simulink model "QAM16"  (R2024a)
settings: Solver=ode45  StartTime=0.0  StopTime=5000  RelTol=1e-3  EnableMultiTasking=on
PreLoadFcn:
  | QAM16_PreLoadFcn
values from neighbouring files (symbols this model uses):
  chan = [1+j*0.1 .2 j*0.2 0 0 0 0 0 0 0]    [QAM16_PreLoadFcn.m]
  hh = sinc(-3:.25:3)    [QAM16_PreLoadFcn.m]
  k = 9    [QAM16_PreLoadFcn.m]
  k_i0 = (4*theta_0*theta_0)/(1+2*eta*theta_0+theta_0*theta_0)    [QAM16_PreLoadFcn.m]
  k_p0 = (4*eta*theta_0)/(1+2*eta*theta_0+theta_0*theta_0)    [QAM16_PreLoadFcn.m]
  mu = 0.004    [QAM16_PreLoadFcn.m]
undefined symbols (not defined in the file or in its folder): j, QAM, S, vsva2197, xcvc1902, xlipgetpartsetting
libraries: hdlBasic x260, dspmlti4 x2, hdlUtilities x1, hdlDSPIP x1, simulink x1, vmcUtilities x1
(part 1 of 3)
settings Model: Creator=alexc  LastModifiedBy=sdegala
settings SolverCC: AlgebraicLoopSolver=TrustRegion
settings DataIOCC: SaveFormat=Array  SignalLoggingSaveFormat=ModelDataLogs  ReturnWorkspaceOutputs=off  SignalLoggingName=sigsOut
settings OptimizationCC: BlockReduction=off  BooleanDataType=off  DefaultParameterBehavior=Inlined  ExpressionDepthLimit=2147483647  InitFltsAndDblsToZero=on  LifeSpan=inf
settings DebuggingCC: SaveWithParameterizedLinksMsg=none  UnderspecifiedInitializationDetection=Classic  MergeDetectMultiDrivingBlocksExec=none  SignalResolutionControl=TryResolveAllWithWarning  MultiTaskDSMMsg=warning  MultiTaskCondExecSysMsg=none  FcnCallInpInsideContextMsg=warning  UnconnectedInputMsg=warning  UnconnectedOutputMsg=warning  UnconnectedLineMsg=warning  StateNameClashWarn=warning  SFUnexpectedBacktrackingDiag=warning  SFNoUnconditionalDefaultTransitionDiag=warning  SFExecutionAtInitializationDiag=none  ArithmeticOperatorsInVariantConditions=warning
settings HardwareCC: ProdBitPerPointer=32  ProdBitPerSizeT=32  ProdBitPerPtrDiffT=32  ProdLargestAtomicFloat=None  ProdIntDivRoundTo=Undefined  ProdEndianess=Unspecified  ProdWordSize=32  ProdHWDeviceType=32-bit Generic  TargetUnknown=on
settings ModelReferenceCC: EnableRefExpFcnMdlSchedulingChecks=on  PropagateSignalLabelsOutOfModel=off
settings SFSimCC: SimUseLocalCustomCode=off  CustomCodeUndefinedFunction=UseInterfaceOnly
settings RTWCC: RTWUseLocalCustomCode=off  GPUComputeCapability=3.5  DLArmComputeVersion=19.05
settings CodeAppCC: StateflowObjectComments=on
settings GRTTargetCC: TargetFcnLib=ansi_tfl_tmw.mat  TargetLangStandard=C89/C90 (ANSI)  CombineOutputUpdateFcns=off  GRTInterface=on
settings ConfigComp: CovMetricSettings=dw  CovSaveCumulativeToWorkspaceVar=on  CovSaveSingleToWorkspaceVar=on  CovExternalEMLEnable=off

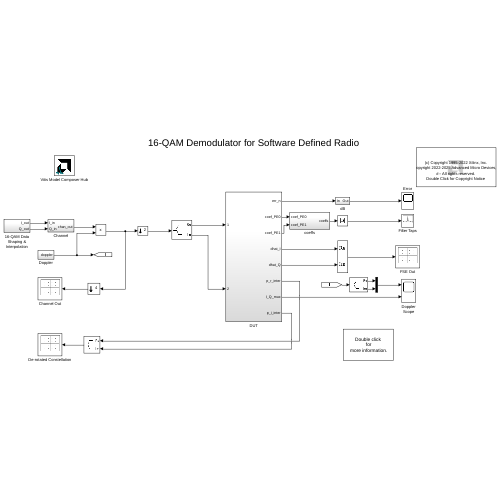
[thumbnail: Simulink's stored preview of the top-level diagram]
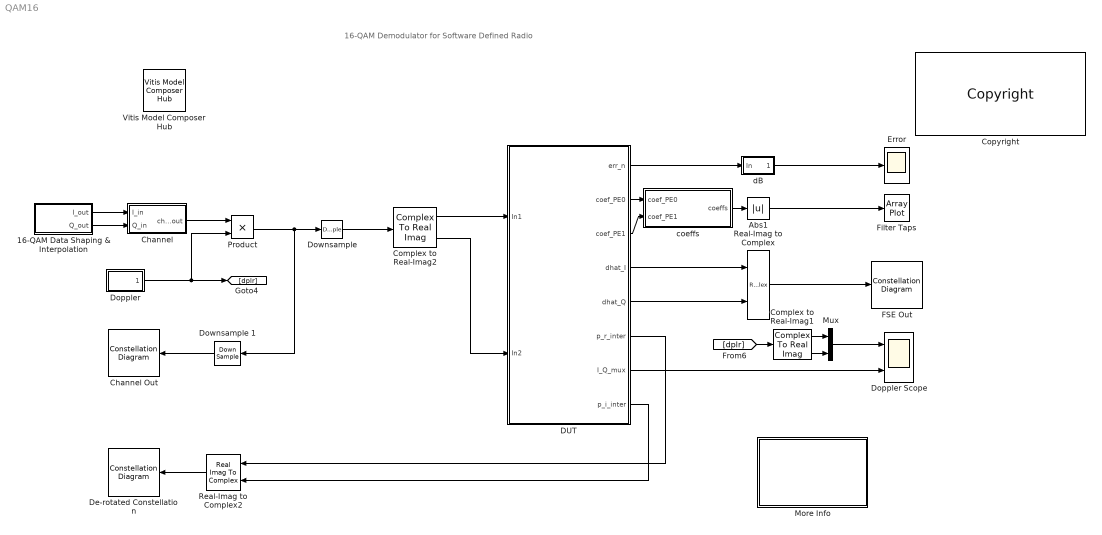
== system QAM16 ==
  note: 16-QAM Demodulator for Software Defined Radio
  16-QAM Data Shaping & Interpolation : Subsystem
  Abs1 : Abs
  Channel : Subsystem
  Channel Out : ConstellationDiagram  WindowPosition=[510.000000,97.000000,342.000000,335.000000,]  Visible=on  ScopeFrameLocation=window  SymbolsToDisplaySource=Property  SymbolsToDisplay=1000  ReferenceConstellation=16-QAM  ShowReferenceConstellation=off  ColorFading=on  DefaultConfigurationName=comm.scopes.ConstellationDiagramBlockCfg
  Complex to Real-Imag1 : ComplexToRealImag
  Complex to Real-Imag2 : ComplexToRealImag
  Copyright : hdlUtilities/Copyright  copyrighttext="(c) Copyright 1995-2022 Xilinx, Inc. <br>(c) Copyright 2022-2025 Advanced Micro Devices, Inc. All rights reserved.<br><br>This document  contains proprietary, confidential information that may be used, copied and/or disclosed only as authorized by a valid licensing agreement with Advanced Micro Devices, Inc. This copyright notice must be retained on all authorized copies.<br><br> This code is provided \"as is\". Advanced Micro Devices, Inc. makes, and the end user receives, no warranties or conditions, express, implied, statutory or otherwise, and Advanced Micro Devices, Inc. specifically disclaims any implied warranties of merchantability, <br>non-infringement, or fitness for a particular purpose."  block_type=copyright
  DUT : Subsystem
  De-rotated Constellation : ConstellationDiagram  WindowPosition=[176.000000,360.000000,339.000000,337.000000,]  Visible=on  ScopeFrameLocation=window  SymbolsToDisplaySource=Property  SymbolsToDisplay=1000  ReferenceConstellation=16-QAM  ColorFading=on  DefaultConfigurationName=comm.scopes.ConstellationDiagramBlockCfg
  Doppler : Subsystem
  Doppler Scope : Scope  NumInputPorts=2
  "Downsample " : DownSample  RateOptions=Allow multirate processing
  Downsample 1 : DownSample  N=4  RateOptions=Allow multirate processing
  Error : Scope
  FSE Out : ConstellationDiagram  WindowPosition=[845.000000,304.000000,340.000000,342.000000,]  Visible=on  ScopeFrameLocation=window  SymbolsToDisplaySource=Property  SymbolsToDisplay=1000  ReferenceConstellation=16-QAM  ShowReferenceConstellation=off  ColorFading=on  DefaultConfigurationName=comm.scopes.ConstellationDiagramBlockCfg
  Filter Taps : ArrayPlot  WindowPosition=[66.000000,260.000000,329.000000,270.000000,]  Visible=on  ScopeFrameLocation=window  PlotType=Line  AxesScaling=Manual  MaximizeAxes=On  XLabel=Samples  YLabel=Filter Coefficients  YLimits=[0.005979,1.0369]  DefaultConfigurationName=dsp.scopes.ArrayPlotBlockSpecification
  More Info : Subsystem
      mask Display: disp('Double click\n for\n more information.')
  Mux : Mux  Inputs=2
  Product : Product  InputSameDT=on  SaturateOnIntegerOverflow=on  OutDataTypeStr=Inherit: Same as first input
  Real-Imag to Complex : RealImagToComplex
  Real-Imag to Complex2 : RealImagToComplex
  Vitis Model Composer Hub : vmcUtilities/Vitis Model Composer Hub  Tag=genX  CodeGeneration=off  SubsystemName=DUT  BlockHierPath=QAM16/DUT  CompilationType=HDLCompilation  SubsystemType=HDLNode  ExportTypeV2=IP Catalog  StartColumn=1  NumberOfColumns=1  TargetDirectory=./netlist  exportDesign=on  analyzeDesign=off  validateDesignOnHw=off  ExportType=System Generator  IpVendor=xilinx.com  IpLibrary=hls  IpVersion=1.0  IpHWLanguage=Verilog  AieCompilerOptions={}  AieSimulatorOptions={}  CreateTestbench=off  TestbenchStackSize=10  RunRtlSim=off  RunCSim=off  RunAieSim=off  AieSimTimeout=50000  RunAieSimProfiling=off  LaunchVitisAnalyzer=off  PlotOutput=off  RunX86Sim=off  X86SimTimeout=10  GenHwImage=off  GenLibadfXo=on  GenHwValidationCode=off  PlatformType=Not Specified  HwSystemType=Baremetal  HwValidationTarget=hw  ProjDevice=xcvc1902-vsva2197-1LP-e-S  ProjDevicePart=xcvc1902-vsva2197-1LP-e-S  AIEType=AIE  SamplePeriod=-1  ClockFrequency=200  DataPathParallelism=1  xilinxfamily=versalaicore  part=xcvc1902  speed=-1LP-e-S  package=vsva2197  directory=./netlist/ip/DUT/src  testbench=off  incr_netlist=off  synthesis_tool=Vivado  clock_wrapper=Clock Enables  dbl_ovrd=According to Block Masks  dcm_input_clock_period=10  sysclk_period=10  simulink_period=1  eval_field=0  IPInfoJsonString="{\"DUTSubsystemName\":\"DUT\",\"HDLSubsystem\":{\"SubsystemName\":\"DUT\",\"IPName\":\"DUT\",\"IPLibrary\":\"VMC\",\"IPVendor\":\"User Company\",\"IPVersion\":\"1.0\",\"TargetDirectory\":\"./netlist\",\"SubsystemDir\":\"./netlist/ip/DUT\",\"FreqHz\":\"100000000\"},\"SubsystemTag\":\"HDLNode\"}"  LogFileName=/proj/xhdhdstaff5/sdegala/Head1/HEAD/ModelComposer_Sept16/Vitis_Model_Composer/Examples/HDL/Digital_Communications/16_QAM_demodulator/netlist/model_composer.log  NThreads=4  IPConfigFile=/tmp/vmctmp-9769773316677438567/QAM16_ipconfig.json
  coeffs : Subsystem
  dB : Subsystem
  wires:
  [dplr] -> Complex to Real-Imag1/1
  Complex to Real-Imag2/1 -> DUT/1(In1)
  Abs1/1 -> Filter Taps/1
  DUT/8(p_i_inter) -> Real-Imag to Complex2/2
  dB/1(Out) -> Error/1
  16-QAM Data Shaping & Interpolation/2(Q_out) -> Channel/2(Q_in)
  Mux/1 -> Doppler Scope/1
  DUT/4(dhat_I) -> Real-Imag to Complex/1
  Channel/1(chan_out) -> Product/1
  DUT/6(p_r_inter) -> Real-Imag to Complex2/1
  Downsample 1/1 -> Channel Out/1
  DUT/1(err_n) -> dB/1(In)
  Real-Imag to Complex2/1 -> De-rotated Constellation/1
  Complex to Real-Imag1/2 -> Mux/2
  16-QAM Data Shaping & Interpolation/1(I_out) -> Channel/1(I_in)
  DUT/5(dhat_Q) -> Real-Imag to Complex/2
  Complex to Real-Imag2/2 -> DUT/2(In2)
  Complex to Real-Imag1/1 -> Mux/1
  Real-Imag to Complex/1 -> FSE Out/1
  Doppler/1(doppler) -> Product/2, [dplr]
  Product/1 -> "Downsample "/1, Downsample 1/1
  "Downsample "/1 -> Complex to Real-Imag2/1
  DUT/7(I_Q_mux) -> Doppler Scope/2
  DUT/2(coef_PE0) -> coeffs/1(coef_PE0)
  coeffs/1(coeffs) -> Abs1/1
  DUT/3(coef_PE1) -> coeffs/2(coef_PE1)

== system QAM16/16-QAM Data Shaping & Interpolation ==
  Complex to Real-Imag5 : ComplexToRealImag
  "FIR Interpolation " : dspmlti4/FIR Interpolation  FilterSource=Dialog parameters  PrivateCoeffs=0  h=[hh]  L=4  FilterObject=Hm_firinterp  framing=Allow multirate processing  outputBufInitCond=0  roundingMode=Floor  overflowMode=off  firstCoeffDataTypeStr=Inherit: Same word length as input  firstCoeffMin=[]  firstCoeffMax=[]  firstCoeffLastDataTypeStr=Inherit: Same word length as input  outputDataTypeStr=Inherit: Same as accumulator  outputMin=[]  outputMax=[]  outputLastDataTypeStr=Inherit: Same as accumulator
  FIR Interpolation 1 : dspmlti4/FIR Interpolation  FilterSource=Dialog parameters  PrivateCoeffs=0  h=[hh]  L=4  FilterObject=Hm_firinterp  framing=Allow multirate processing  outputBufInitCond=0  roundingMode=Floor  overflowMode=off  firstCoeffDataTypeStr=Inherit: Same word length as input  firstCoeffMin=[]  firstCoeffMax=[]  firstCoeffLastDataTypeStr=Inherit: Same word length as input  outputDataTypeStr=Inherit: Same as accumulator  outputMin=[]  outputMax=[]  outputLastDataTypeStr=Inherit: Same as accumulator
  QAM16 Source : Subsystem
  I_out : Outport  VectorParamsAs1DForOutWhenUnconnected=off
  Q_out : Outport  Port=2  VectorParamsAs1DForOutWhenUnconnected=off
  wires:
  Complex to Real-Imag5/1 -> "FIR Interpolation "/1
  Complex to Real-Imag5/2 -> FIR Interpolation 1/1
  QAM16 Source/1(random_data) -> Complex to Real-Imag5/1
  "FIR Interpolation "/1 -> I_out/1
  FIR Interpolation 1/1 -> Q_out/1

== system QAM16/Channel ==
  I_in : Inport
  Q_in : Inport  Port=2
  Channel : Subsystem
  Channel1 : Subsystem
  Gain : Gain  Gain=j  SaturateOnIntegerOverflow=on  OutDataTypeStr=Inherit: Same as input  ParamDataTypeStr=Inherit: Same as input
  Sum : Sum  InputSameDT=on  SaturateOnIntegerOverflow=on  OutDataTypeStr=Inherit: Same as first input
  chan_out : Outport  VectorParamsAs1DForOutWhenUnconnected=off
  wires:
  Gain/1 -> Sum/2
  Channel/1(y_n) -> Sum/1
  Channel1/1(y_n) -> Gain/1
  I_in/1 -> Channel/1(x_n)
  Q_in/1 -> Channel1/1(x_n)
  Sum/1 -> chan_out/1

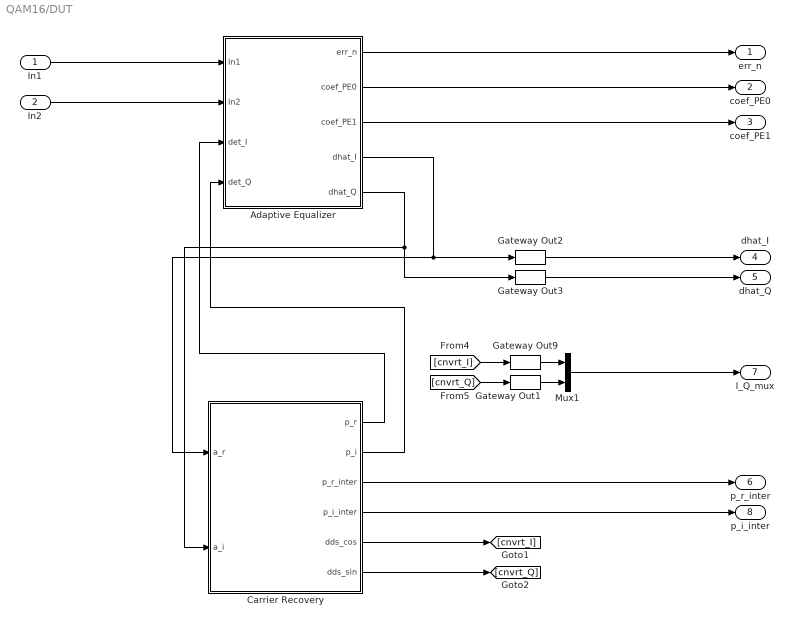
== system QAM16/DUT ==
  In1 : Inport
  In2 : Inport  Port=2
  Adaptive Equalizer : Subsystem
  Carrier Recovery : Subsystem
  Gateway Out{1..3,9} (4 alike) : hdlBasic/Gateway Out  inherit_from_input=off  bool_to_boolean=off  hdl_port=off  rows=1  columns=1  UseAsDAC=off  DACChannel='1'  interface=None  automatic_assignment=on  address_offset=hex2dec('00')  intf_name=''  intf_description=''  timing_constraint=None  locs_specified=off  LOCs={}  io_standard={}  XmcBlockStatus=1  maskContainerNames=group4  block_type=gatewayout  block_config=sysgen:gateway_out_config  block_width_w=590  block_height_w=620  block_width=620  block_height=750
  Mux1 : Mux  Inputs=2
  err_n : Outport
  coef_PE0 : Outport  Port=2
  coef_PE1 : Outport  Port=3
  dhat_I : Outport  Port=4
  dhat_Q : Outport  Port=5
  p_r_inter : Outport  Port=6
  I_Q_mux : Outport  Port=7
  p_i_inter : Outport  Port=8
  wires:
  In1/1 -> Adaptive Equalizer/1(In1)
  Gateway Out1/1 -> Mux1/2
  Carrier Recovery/4(p_i_inter) -> p_i_inter/1
  Adaptive Equalizer/2(coef_PE0) -> coef_PE0/1
  Adaptive Equalizer/1(err_n) -> err_n/1
  In2/1 -> Adaptive Equalizer/2(In2)
  Gateway Out3/1 -> dhat_Q/1
  Mux1/1 -> I_Q_mux/1
  Carrier Recovery/2(p_i) -> Adaptive Equalizer/4(det_Q)
  Carrier Recovery/5(dds_cos) -> [cnvrt_I]
  Adaptive Equalizer/5(dhat_Q) -> Gateway Out3/1, Carrier Recovery/2(a_i)
  Carrier Recovery/3(p_r_inter) -> p_r_inter/1
  Gateway Out9/1 -> Mux1/1
  [cnvrt_Q] -> Gateway Out1/1
  Carrier Recovery/6(dds_sin) -> [cnvrt_Q]
  Adaptive Equalizer/4(dhat_I) -> Gateway Out2/1, Carrier Recovery/1(a_r)
  [cnvrt_I] -> Gateway Out9/1
  Carrier Recovery/1(p_r) -> Adaptive Equalizer/3(det_I)
  Gateway Out2/1 -> dhat_I/1
  Adaptive Equalizer/3(coef_PE1) -> coef_PE1/1

== system QAM16/Doppler ==
  DSP Constant : Constant  VectorParams1D=off  SampleTime=1
  Frequency Delta : simulink/Math Operations/Slider Gain  gain=0.001  low=-0.1  high=0.1
  R:I : RealImagToComplex
  TX Doppler : Subsystem
  Terminator : Terminator
  doppler : Outport  VectorParamsAs1DForOutWhenUnconnected=off
  wires:
  TX Doppler/1(Cos) -> R:I/1
  TX Doppler/2(Sin) -> R:I/2
  Frequency Delta/1 -> TX Doppler/1(In1)
  DSP Constant/1 -> Frequency Delta/1
  R:I/1 -> doppler/1
  TX Doppler/3(DDS Theta) -> Terminator/1

== system QAM16/More Info ==
  note: 16-QAM Demodulator for Software Defined Radio
  note: This design implements an equalized 16-QAM demodulator for use in a software defined
      | radio.  The receiver architecture provides subsystems that demonstrate adaptive channel
      | equalization and carrier tracking on a random QAM data source.
      |
      | In addition to Vitis Model Composer demodulator components, the model includes Simulink
      | subsystems that introduce channel effects and Doppler content into the data source.  Scopes
      | are provided at important nodes for analysis purposes.  The operation of receiver is best
      | illustrated with a long simulation duration, so that the points in the de-rotated constellation
      | have sufficient time to converge.
      |
      | Additional information on software radios can be found at:
      |
      | Chris H. Dick, "Design and implementation of high-performance FPGA signal processing
      | datapaths for software-defined radios" VMEbus Systems, August 2001

== system QAM16/coeffs ==
  note: The equalizer ALU divides the processing between two
      | polyphase arms.  each with their own PE.  The four filter
      | operations are scheduled onto a single complex multiply
      | -accumulate (MAC) engine.  Similarly, the 4 coefficient
      | updates are folded onto a single LMS PE.
  coef_PE0 : Inport
  coef_PE1 : Inport  Port=2
  Buffer : Buffer  N=8
  Discrete Pulse Generator : DiscretePulseGenerator  SampleTime=.5
  Switch1 : Switch  Threshold=.5
  coeffs : Outport
  wires:
  coef_PE0/1 -> Switch1/3
  coef_PE1/1 -> Switch1/1
  Discrete Pulse Generator/1 -> Switch1/2
  Switch1/1 -> Buffer/1
  Buffer/1 -> coeffs/1

== system QAM16/dB ==
  In : Inport
  Abs : Abs
  Constant : Constant  Value=0
  Constant1 : Constant
  Constant2 : Constant
  Gain1 : Gain  Gain=20  SaturateOnIntegerOverflow=on  OutDataTypeStr=Inherit: Same as input  ParamDataTypeStr=Inherit: Same as input
  Multiport Switch : MultiPortSwitch  Inputs=2
  Relational Operator : RelationalOperator  Operator===
  Sum : Sum  Inputs=|++  InputSameDT=on  SaturateOnIntegerOverflow=on  OutDataTypeStr=Inherit: Same as first input
  log10 : Math  Operator=log10  SignedPower=on
  Out : Outport  VectorParamsAs1DForOutWhenUnconnected=off
  wires:
  Multiport Switch/1 -> log10/1
  Constant1/1 -> Multiport Switch/3
  Constant/1 -> Relational Operator/1
  Abs/1 -> Multiport Switch/2, Relational Operator/2
  Constant2/1 -> Sum/2
  Sum/1 -> Multiport Switch/1
  Relational Operator/1 -> Sum/1
  Gain1/1 -> Out/1
  In/1 -> Abs/1
  log10/1 -> Gain1/1

== system QAM16/16-QAM Data Shaping & Interpolation/QAM16 Source ==
  QAM16 - I : Subsystem
  QAM16 -Q : Subsystem
  Real-Imag to Complex : RealImagToComplex
  random_data : Outport  VectorParamsAs1DForOutWhenUnconnected=off
  wires:
  Real-Imag to Complex/1 -> random_data/1
  QAM16 -Q/1(Q) -> Real-Imag to Complex/2
  QAM16 - I/1(I) -> Real-Imag to Complex/1

== system QAM16/Channel/Channel ==
  x_n : Inport
  Channel Response : Subsystem
  y_n : Outport  VectorParamsAs1DForOutWhenUnconnected=off
  wires:
  Channel Response/1(y_n) -> y_n/1
  x_n/1 -> Channel Response/1(x_n)

== system QAM16/Channel/Channel1 ==
  x_n : Inport
  Channel Response : Subsystem
  y_n : Outport  VectorParamsAs1DForOutWhenUnconnected=off
  wires:
  Channel Response/1(y_n) -> y_n/1
  x_n/1 -> Channel Response/1(x_n)

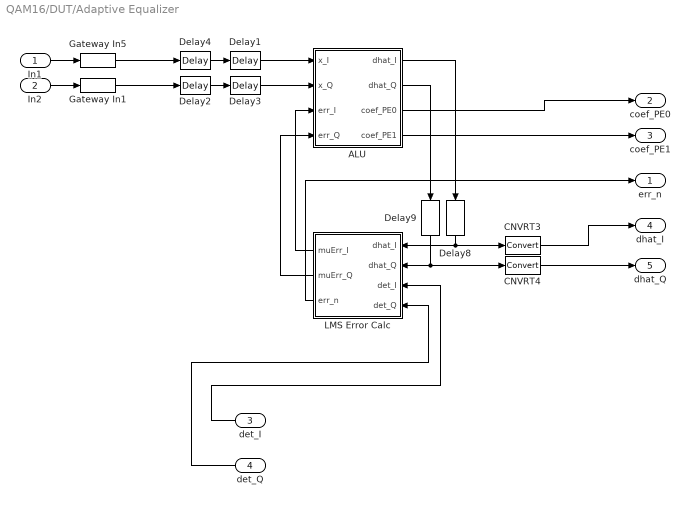
== system QAM16/DUT/Adaptive Equalizer ==
  In1 : Inport
  In2 : Inport  Port=2
  det_I : Inport  Port=3
  det_Q : Inport  Port=4
  ALU : Subsystem
  CNVRT3 : hdlBasic/Convert  gui_display_data_type=Fixed-point  arith_type=Signed (2's comp)  n_bits=18  bin_pt=14  float_type=Single  exp_bits=8  fraction_bits=24  quantization="Round  (unbiased: +/- Inf)"  overflow=Wrap  en=off  latency=0  pipeline=off  XmcBlockStatus=1  maskContainerNames=group2  block_type=convert  block_config=sysgen:Convert_config  block_width=595  block_height=885
  CNVRT4 : hdlBasic/Convert  gui_display_data_type=Fixed-point  arith_type=Signed (2's comp)  n_bits=18  bin_pt=14  float_type=Single  exp_bits=8  fraction_bits=24  quantization="Round  (unbiased: +/- Inf)"  overflow=Wrap  en=off  latency=0  pipeline=off  XmcBlockStatus=1  maskContainerNames=group2  block_type=convert  block_config=sysgen:Convert_config  block_width=595  block_height=885
  Delay{1..4} (4 alike) : hdlBasic/Delay  rst=off  en=off  latency=1  reg_retiming=off  XmcBlockStatus=1  maskContainerNames=group1  block_type=delay  block_config=sysgen:Delay_config
  Delay8 : hdlBasic/Delay  rst=off  en=off  latency=k-7  reg_retiming=off  XmcBlockStatus=1  maskContainerNames=group1  block_type=delay  block_config=sysgen:Delay_config
  Delay9 : hdlBasic/Delay  rst=off  en=off  latency=k-7  reg_retiming=off  XmcBlockStatus=1  maskContainerNames=group1  block_type=delay  block_config=sysgen:Delay_config
  Gateway In1 : hdlBasic/Gateway In  gui_display_data_type=Fixed-point  arith_type=Signed (2's comp)  n_bits=xn_ni  bin_pt=xn_nf  preci_type=Single  exp_width=8  frac_width=24  rows=1  columns=1  quantization="Round  (unbiased: +/- Inf)"  overflow=Saturate  period=2  UseAsADC=off  ADCChannel='1'  interface=None  automatic_assignment=on  address_offset=hex2dec('00')  intf_name=''  intf_description=''  default_value=0  timing_constraint=None  locs_specified=off  LOCs={}  io_standard={}  inherit_from_input=off  hdl_port=on  XmcBlockStatus=1  maskContainerNames=group4  block_type=gatewayin  block_config=sysgen:gateway_in_config  block_width_w=590  block_height_w=620  block_width=640  block_height=850
  Gateway In5 : hdlBasic/Gateway In  gui_display_data_type=Fixed-point  arith_type=Signed (2's comp)  n_bits=xn_ni  bin_pt=xn_nf  preci_type=Single  exp_width=8  frac_width=24  rows=1  columns=1  quantization="Round  (unbiased: +/- Inf)"  overflow=Saturate  period=2  UseAsADC=off  ADCChannel='1'  interface=None  automatic_assignment=on  address_offset=hex2dec('00')  intf_name=''  intf_description=''  default_value=0  timing_constraint=None  locs_specified=off  LOCs={}  io_standard={}  inherit_from_input=off  hdl_port=on  XmcBlockStatus=1  maskContainerNames=group4  block_type=gatewayin  block_config=sysgen:gateway_in_config  block_width_w=590  block_height_w=620  block_width=640  block_height=850
  LMS Error Calc : Subsystem
  err_n : Outport
  coef_PE0 : Outport  Port=2
  coef_PE1 : Outport  Port=3
  dhat_I : Outport  Port=4
  dhat_Q : Outport  Port=5
  wires:
  ALU/2(dhat_Q) -> Delay9/1
  ALU/3(coef_PE0) -> coef_PE0/1
  det_I/1 -> LMS Error Calc/3(det_I)
  LMS Error Calc/3(err_n) -> err_n/1
  Delay9/1 -> LMS Error Calc/2(dhat_Q), CNVRT4/1
  In2/1 -> Gateway In1/1
  det_Q/1 -> LMS Error Calc/4(det_Q)
  CNVRT3/1 -> dhat_I/1
  In1/1 -> Gateway In5/1
  Delay2/1 -> Delay3/1
  Delay3/1 -> ALU/2(x_Q)
  Gateway In5/1 -> Delay4/1
  ALU/1(dhat_I) -> Delay8/1
  Delay8/1 -> LMS Error Calc/1(dhat_I), CNVRT3/1
  Delay1/1 -> ALU/1(x_I)
  LMS Error Calc/2(muErr_Q) -> ALU/4(err_Q)
  LMS Error Calc/1(muErr_I) -> ALU/3(err_I)
  CNVRT4/1 -> dhat_Q/1
  Gateway In1/1 -> Delay2/1
  Delay4/1 -> Delay1/1
  ALU/4(coef_PE1) -> coef_PE1/1

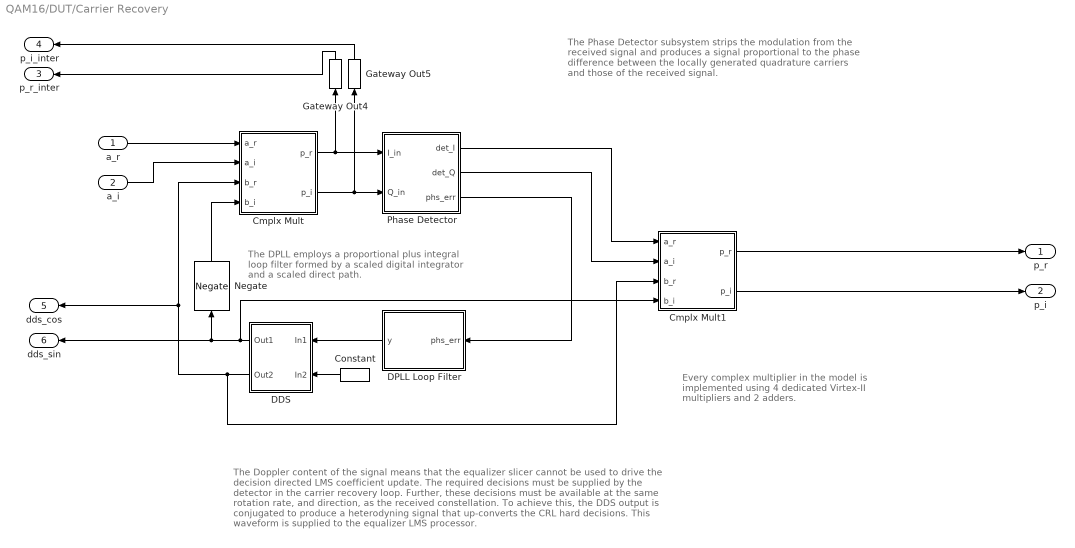
== system QAM16/DUT/Carrier Recovery ==
  note: The DPLL employs a proportional plus integral
      | loop filter formed by a scaled digital integrator
      | and a scaled direct path.
  note: The Phase Detector subsystem strips the modulation
      | from the received signal and produces a signal proportional
      | to the phase difference between the locally generated
      | quadrature carriers and those of the received signal.
  note: The Doppler content of the signal means that the equalizer slicer cannot be used
      | to drive the decision directed LMS coefficient update.  The required decisions must
      | be supplied by the detector in the carrier recovery loop.  Further, these decisions
      | must be available at the same rotation rate, and direction, as the received constellation.
      | To achieve this, the DDS output is conjugated to produce a heterodyning signal
      | that up-converts the CRL hard decisions. This waveform is supplied to the equalizer
      | LMS processor.
  note: Every complex multiplier in the model is
      | implemented using 4 dedicated Virtex-II
      | multipliers and 2 adders.
  a_r : Inport
  a_i : Inport  Port=2
  Cmplx Mult : Subsystem
  Cmplx Mult1 : Subsystem
  Constant : hdlBasic/Constant  const=1  gui_display_data_type=Boolean  arith_type=Boolean  n_bits=1  bin_pt=0  preci_type=Single  exp_width=8  frac_width=24  explicit_period=off  period=1  XmcBlockStatus=1  maskContainerNames=tabcontainer1  block_type=constant  block_config=sysgen:Constant_config
  DDS : Subsystem
  DPLL Loop Filter : Subsystem
  Gateway Out4 : hdlBasic/Gateway Out  inherit_from_input=off  bool_to_boolean=off  hdl_port=on  rows=1  columns=1  UseAsDAC=off  DACChannel='1'  interface=None  automatic_assignment=on  address_offset=hex2dec('00')  intf_name=''  intf_description=''  timing_constraint="Data Rate;  Set 'FAST' Attribute"  locs_specified=off  LOCs={}  io_standard={}  XmcBlockStatus=1  maskContainerNames=group4  block_type=gatewayout  block_config=sysgen:gateway_out_config  block_width_w=590  block_height_w=620  block_width=620  block_height=750
  Gateway Out5 : hdlBasic/Gateway Out  inherit_from_input=off  bool_to_boolean=off  hdl_port=on  rows=1  columns=1  UseAsDAC=off  DACChannel='1'  interface=None  automatic_assignment=on  address_offset=hex2dec('00')  intf_name=''  intf_description=''  timing_constraint="Data Rate;  Set 'FAST' Attribute"  locs_specified=off  LOCs={}  io_standard={}  XmcBlockStatus=1  maskContainerNames=group4  block_type=gatewayout  block_config=sysgen:gateway_out_config  block_width_w=590  block_height_w=620  block_width=620  block_height=750
  Negate : hdlBasic/Negate  precision=Full  arith_type=Unsigned  n_bits=8  bin_pt=2  quantization=Truncate  overflow=Wrap  en=off  latency=0  XmcBlockStatus=1  maskContainerNames=tabcontainer1  block_type=negate  block_config=sysgen:Negate_config
  Phase Detector : Subsystem
  p_r : Outport
  p_i : Outport  Port=2
  p_r_inter : Outport  Port=3
  p_i_inter : Outport  Port=4
  dds_cos : Outport  Port=5
  dds_sin : Outport  Port=6
  wires:
  DPLL Loop Filter/1(y) -> DDS/1(In1)
  Negate/1 -> Cmplx Mult/4(b_i)
  Cmplx Mult/1(p_r) -> Gateway Out4/1, Phase Detector/1(I_in)
  Cmplx Mult1/2(p_i) -> p_i/1
  a_r/1 -> Cmplx Mult/1(a_r)
  DDS/2(Out2) -> dds_cos/1, Cmplx Mult/3(b_r), Cmplx Mult1/3(b_r)
  Gateway Out5/1 -> p_i_inter/1
  Constant/1 -> DDS/2(In2)
  a_i/1 -> Cmplx Mult/2(a_i)
  DDS/1(Out1) -> Negate/1, dds_sin/1, Cmplx Mult1/4(b_i)
  Cmplx Mult1/1(p_r) -> p_r/1
  Phase Detector/3(phs_err) -> DPLL Loop Filter/1(phs_err)
  Phase Detector/2(det_Q) -> Cmplx Mult1/2(a_i)
  Cmplx Mult/2(p_i) -> Gateway Out5/1, Phase Detector/2(Q_in)
  Phase Detector/1(det_I) -> Cmplx Mult1/1(a_r)
  Gateway Out4/1 -> p_r_inter/1

== system QAM16/Doppler/TX Doppler ==
  In1 : Inport
  Sum5 : Sum  Inputs=|++  InputSameDT=on  SaturateOnIntegerOverflow=on  OutDataTypeStr=Inherit: Same as first input
  Trigonometric Function1 : Trigonometry  Operator=cos
  Trigonometric Function2 : Trigonometry
  Unit Delay2 : UnitDelay  HasFrameUpgradeWarning=on
  c2 : Gain  Gain=2*pi  SaturateOnIntegerOverflow=on  OutDataTypeStr=Inherit: Same as input  ParamDataTypeStr=Inherit: Same as input
  c3 : Gain  SaturateOnIntegerOverflow=on  OutDataTypeStr=Inherit: Same as input  ParamDataTypeStr=Inherit: Same as input
  Cos : Outport  VectorParamsAs1DForOutWhenUnconnected=off
  Sin : Outport  Port=2  VectorParamsAs1DForOutWhenUnconnected=off
  DDS Theta : Outport  Port=3  VectorParamsAs1DForOutWhenUnconnected=off
  wires:
  c2/1 -> Trigonometric Function1/1, Trigonometric Function2/1, DDS Theta/1
  Sum5/1 -> Unit Delay2/1
  Unit Delay2/1 -> c2/1, Sum5/2
  Trigonometric Function2/1 -> c3/1
  c3/1 -> Sin/1
  Trigonometric Function1/1 -> Cos/1
  In1/1 -> Sum5/1

== system QAM16/16-QAM Data Shaping & Interpolation/QAM16 Source/QAM16 - I ==
  Constant : Constant  Value=3
  Gain : Gain  Gain=2  SaturateOnIntegerOverflow=on  OutDataTypeStr=Inherit: Same as input  ParamDataTypeStr=Inherit: Same as input
  Gain1 : Gain  Gain=1/3  SaturateOnIntegerOverflow=on  OutDataTypeStr=Inherit: Same as input  ParamDataTypeStr=Inherit: Same as input
  Random Integer Generator : Subsystem  mask{M=4, seed=11, Ts=4}
      mask prompts: M "M-ary Number"; seed "Initial seed"; Ts "Sample Time"
  Sum : Sum  Inputs=|+-  InputSameDT=on  SaturateOnIntegerOverflow=on  OutDataTypeStr=Inherit: Same as first input
  I : Outport  VectorParamsAs1DForOutWhenUnconnected=off
  wires:
  Gain1/1 -> I/1
  Sum/1 -> Gain1/1
  Constant/1 -> Sum/2
  Gain/1 -> Sum/1
  Random Integer Generator/1(Out1) -> Gain/1

== system QAM16/16-QAM Data Shaping & Interpolation/QAM16 Source/QAM16 -Q ==
  Constant : Constant  Value=3
  Gain : Gain  Gain=2  SaturateOnIntegerOverflow=on  OutDataTypeStr=Inherit: Same as input  ParamDataTypeStr=Inherit: Same as input
  Gain1 : Gain  Gain=1/3  SaturateOnIntegerOverflow=on  OutDataTypeStr=Inherit: Same as input  ParamDataTypeStr=Inherit: Same as input
  Random Integer Generator : Subsystem  mask{M=4, seed=72, Ts=4}
      mask prompts: M "M-ary Number"; seed "Initial seed"; Ts "Sample Time"
  Sum : Sum  Inputs=|+-  InputSameDT=on  SaturateOnIntegerOverflow=on  OutDataTypeStr=Inherit: Same as first input
  Q : Outport  VectorParamsAs1DForOutWhenUnconnected=off
  wires:
  Gain1/1 -> Q/1
  Sum/1 -> Gain1/1
  Constant/1 -> Sum/2
  Gain/1 -> Sum/1
  Random Integer Generator/1(Out1) -> Gain/1

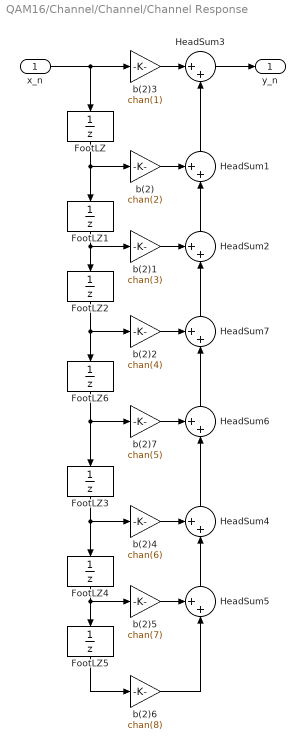
== system QAM16/Channel/Channel/Channel Response ==
  x_n : Inport
  FootLZ : UnitDelay  HasFrameUpgradeWarning=on
  FootLZ{1..2,4..6} (5 alike) : UnitDelay  SampleTime=-1  HasFrameUpgradeWarning=on
  FootLZ3 : UnitDelay  HasFrameUpgradeWarning=on
  HeadSum{1..2,4..7} (6 alike) : Sum  Inputs=++|  InputSameDT=on  SaturateOnIntegerOverflow=on  OutDataTypeStr=Inherit: Same as first input
  HeadSum3 : Sum  Inputs=|++  InputSameDT=on  SaturateOnIntegerOverflow=on  OutDataTypeStr=Inherit: Same as first input
  b(2) : Gain  Gain=chan(2)  SaturateOnIntegerOverflow=on  OutDataTypeStr=Inherit: Same as input  ParamDataTypeStr=Inherit: Same as input
  b(2)1 : Gain  Gain=chan(3)  SaturateOnIntegerOverflow=on  OutDataTypeStr=Inherit: Same as input  ParamDataTypeStr=Inherit: Same as input
  b(2)2 : Gain  Gain=chan(4)  SaturateOnIntegerOverflow=on  OutDataTypeStr=Inherit: Same as input  ParamDataTypeStr=Inherit: Same as input
  b(2)3 : Gain  Gain=chan(1)  SaturateOnIntegerOverflow=on  OutDataTypeStr=Inherit: Same as input  ParamDataTypeStr=Inherit: Same as input
  b(2)4 : Gain  Gain=chan(6)  SaturateOnIntegerOverflow=on  OutDataTypeStr=Inherit: Same as input  ParamDataTypeStr=Inherit: Same as input
  b(2)5 : Gain  Gain=chan(7)  SaturateOnIntegerOverflow=on  OutDataTypeStr=Inherit: Same as input  ParamDataTypeStr=Inherit: Same as input
  b(2)6 : Gain  Gain=chan(8)  SaturateOnIntegerOverflow=on  OutDataTypeStr=Inherit: Same as input  ParamDataTypeStr=Inherit: Same as input
  b(2)7 : Gain  Gain=chan(5)  SaturateOnIntegerOverflow=on  OutDataTypeStr=Inherit: Same as input  ParamDataTypeStr=Inherit: Same as input
  y_n : Outport  VectorParamsAs1DForOutWhenUnconnected=off
  wires:
  HeadSum3/1 -> y_n/1
  HeadSum1/1 -> HeadSum3/2
  b(2)3/1 -> HeadSum3/1
  x_n/1 -> b(2)3/1, FootLZ/1
  HeadSum2/1 -> HeadSum1/2
  b(2)1/1 -> HeadSum2/1
  b(2)/1 -> HeadSum1/1
  FootLZ1/1 -> b(2)1/1, FootLZ2/1
  FootLZ/1 -> FootLZ1/1, b(2)/1
  FootLZ2/1 -> b(2)2/1, FootLZ6/1
  b(2)7/1 -> HeadSum6/1
  b(2)6/1 -> HeadSum5/2
  HeadSum5/1 -> HeadSum4/2
  b(2)5/1 -> HeadSum5/1
  b(2)4/1 -> HeadSum4/1
  FootLZ5/1 -> b(2)6/1
  FootLZ4/1 -> b(2)5/1, FootLZ5/1
  FootLZ3/1 -> FootLZ4/1, b(2)4/1
  FootLZ6/1 -> b(2)7/1, FootLZ3/1
  b(2)2/1 -> HeadSum7/1
  HeadSum7/1 -> HeadSum2/2
  HeadSum4/1 -> HeadSum6/2
  HeadSum6/1 -> HeadSum7/2

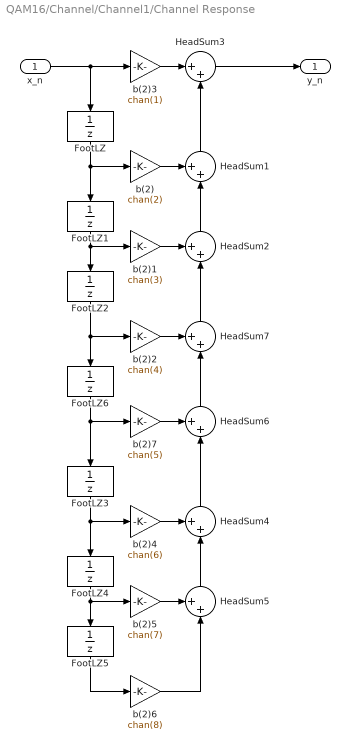
== system QAM16/Channel/Channel1/Channel Response ==
  x_n : Inport
  FootLZ : UnitDelay  HasFrameUpgradeWarning=on
  FootLZ{1..2,4..6} (5 alike) : UnitDelay  SampleTime=-1  HasFrameUpgradeWarning=on
  FootLZ3 : UnitDelay  HasFrameUpgradeWarning=on
  HeadSum{1..2,4..7} (6 alike) : Sum  Inputs=++|  InputSameDT=on  SaturateOnIntegerOverflow=on  OutDataTypeStr=Inherit: Same as first input
  HeadSum3 : Sum  Inputs=|++  InputSameDT=on  SaturateOnIntegerOverflow=on  OutDataTypeStr=Inherit: Same as first input
  b(2) : Gain  Gain=chan(2)  SaturateOnIntegerOverflow=on  OutDataTypeStr=Inherit: Same as input  ParamDataTypeStr=Inherit: Same as input
  b(2)1 : Gain  Gain=chan(3)  SaturateOnIntegerOverflow=on  OutDataTypeStr=Inherit: Same as input  ParamDataTypeStr=Inherit: Same as input
  b(2)2 : Gain  Gain=chan(4)  SaturateOnIntegerOverflow=on  OutDataTypeStr=Inherit: Same as input  ParamDataTypeStr=Inherit: Same as input
  b(2)3 : Gain  Gain=chan(1)  SaturateOnIntegerOverflow=on  OutDataTypeStr=Inherit: Same as input  ParamDataTypeStr=Inherit: Same as input
  b(2)4 : Gain  Gain=chan(6)  SaturateOnIntegerOverflow=on  OutDataTypeStr=Inherit: Same as input  ParamDataTypeStr=Inherit: Same as input
  b(2)5 : Gain  Gain=chan(7)  SaturateOnIntegerOverflow=on  OutDataTypeStr=Inherit: Same as input  ParamDataTypeStr=Inherit: Same as input
  b(2)6 : Gain  Gain=chan(8)  SaturateOnIntegerOverflow=on  OutDataTypeStr=Inherit: Same as input  ParamDataTypeStr=Inherit: Same as input
  b(2)7 : Gain  Gain=chan(5)  SaturateOnIntegerOverflow=on  OutDataTypeStr=Inherit: Same as input  ParamDataTypeStr=Inherit: Same as input
  y_n : Outport  VectorParamsAs1DForOutWhenUnconnected=off
  wires:
  HeadSum3/1 -> y_n/1
  HeadSum1/1 -> HeadSum3/2
  b(2)3/1 -> HeadSum3/1
  x_n/1 -> b(2)3/1, FootLZ/1
  HeadSum2/1 -> HeadSum1/2
  b(2)1/1 -> HeadSum2/1
  b(2)/1 -> HeadSum1/1
  FootLZ1/1 -> b(2)1/1, FootLZ2/1
  FootLZ/1 -> FootLZ1/1, b(2)/1
  HeadSum4/1 -> HeadSum6/2
  b(2)7/1 -> HeadSum6/1
  b(2)6/1 -> HeadSum5/2
  HeadSum5/1 -> HeadSum4/2
  b(2)5/1 -> HeadSum5/1
  b(2)4/1 -> HeadSum4/1
  FootLZ5/1 -> b(2)6/1
  FootLZ4/1 -> b(2)5/1, FootLZ5/1
  FootLZ3/1 -> FootLZ4/1, b(2)4/1
  FootLZ2/1 -> b(2)2/1, FootLZ6/1
  FootLZ6/1 -> FootLZ3/1, b(2)7/1
  HeadSum6/1 -> HeadSum7/2
  HeadSum7/1 -> HeadSum2/2
  b(2)2/1 -> HeadSum7/1

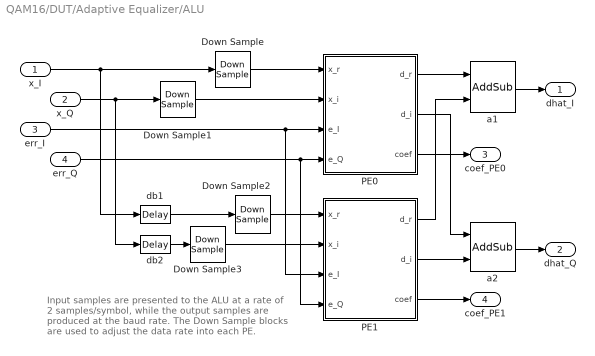
== system QAM16/DUT/Adaptive Equalizer/ALU ==
  note: Input samples are presented to the ALU at a rate
      | of 2 samples/symbol, while the output samples
      | are produced at the baud rate.  The Down
      | Sample blocks are used to adjust the data rate
      | into each PE.
  x_I : Inport
  x_Q : Inport  Port=2
  err_I : Inport  Port=3
  err_Q : Inport  Port=4
  Down Sample{,1..3} (4 alike) : hdlBasic/Down Sample  sample_ratio=2  sample_phase="Last Value of Frame  (most efficient)"  en=off  rst=off  latency=2  XmcBlockStatus=1  maskContainerNames=group1  block_type=dsamp  block_config=sysgen:Downsample_config
  PE0 : Subsystem
  PE1 : Subsystem
  a1 : hdlBasic/AddSub  mode=Addition  use_carryin=off  use_carryout=off  en=off  latency=2  precision=User Defined  arith_type="Signed  (2's comp)"  n_bits=24  bin_pt=20  quantization=Truncate  overflow=Saturate  use_behavioral_HDL=on  hw_selection=Fabric  pipelined=off  use_rpm=off  XmcBlockStatus=1  maskContainerNames=tabcontainer1  block_type=addsub  block_config=sysgen:Addsub_config
  a2 : hdlBasic/AddSub  mode=Addition  use_carryin=off  use_carryout=off  en=off  latency=2  precision=User Defined  arith_type="Signed  (2's comp)"  n_bits=24  bin_pt=20  quantization=Truncate  overflow=Saturate  use_behavioral_HDL=on  hw_selection=Fabric  pipelined=off  use_rpm=off  XmcBlockStatus=1  maskContainerNames=tabcontainer1  block_type=addsub  block_config=sysgen:Addsub_config
  db1 : hdlBasic/Delay  rst=off  en=off  latency=1  reg_retiming=off  XmcBlockStatus=1  maskContainerNames=group1  block_type=delay  block_config=sysgen:Delay_config
  db2 : hdlBasic/Delay  rst=off  en=off  latency=1  reg_retiming=off  XmcBlockStatus=1  maskContainerNames=group1  block_type=delay  block_config=sysgen:Delay_config
  dhat_I : Outport  VectorParamsAs1DForOutWhenUnconnected=off
  dhat_Q : Outport  Port=2  VectorParamsAs1DForOutWhenUnconnected=off
  coef_PE0 : Outport  Port=3  VectorParamsAs1DForOutWhenUnconnected=off
  coef_PE1 : Outport  Port=4  VectorParamsAs1DForOutWhenUnconnected=off
  wires:
  err_I/1 -> PE0/3(e_I), PE1/3(e_I)
  err_Q/1 -> PE0/4(e_Q), PE1/4(e_Q)
  x_I/1 -> db1/1, Down Sample/1
  x_Q/1 -> Down Sample1/1, db2/1
  Down Sample1/1 -> PE0/2(x_i)
  PE0/1(d_r) -> a1/1
  PE0/2(d_i) -> a2/1
  a1/1 -> dhat_I/1
  a2/1 -> dhat_Q/1
  db1/1 -> Down Sample2/1
  db2/1 -> Down Sample3/1
  PE0/3(coef) -> coef_PE0/1
  Down Sample2/1 -> PE1/1(x_r)
  Down Sample3/1 -> PE1/2(x_i)
  PE1/3(coef) -> coef_PE1/1
  PE1/1(d_r) -> a1/2
  PE1/2(d_i) -> a2/2
  Down Sample/1 -> PE0/1(x_r)

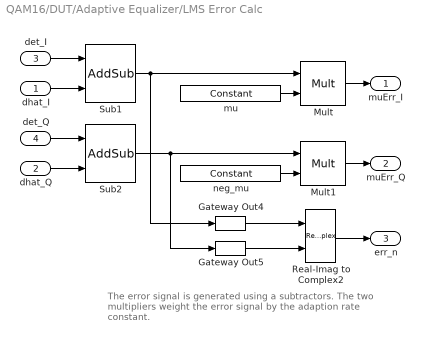
== system QAM16/DUT/Adaptive Equalizer/LMS Error Calc ==
  note: The error signal is generated using a subtractors.  The
      | two multipliers weight  the error signal by the adaption
      | rate constant.
  dhat_I : Inport
  dhat_Q : Inport  Port=2
  det_I : Inport  Port=3
  det_Q : Inport  Port=4
  Gateway Out4 : hdlBasic/Gateway Out  inherit_from_input=off  bool_to_boolean=off  hdl_port=off  rows=1  columns=1  UseAsDAC=off  DACChannel='1'  interface=None  automatic_assignment=on  address_offset=hex2dec('00')  intf_name=''  intf_description=''  timing_constraint=None  locs_specified=off  LOCs={}  io_standard={}  XmcBlockStatus=1  maskContainerNames=group4  block_type=gatewayout  block_config=sysgen:gateway_out_config  block_width_w=590  block_height_w=620  block_width=620  block_height=750
  Gateway Out5 : hdlBasic/Gateway Out  inherit_from_input=off  bool_to_boolean=off  hdl_port=off  rows=1  columns=1  UseAsDAC=off  DACChannel='1'  interface=None  automatic_assignment=on  address_offset=hex2dec('00')  intf_name=''  intf_description=''  timing_constraint=None  locs_specified=off  LOCs={}  io_standard={}  XmcBlockStatus=1  maskContainerNames=group4  block_type=gatewayout  block_config=sysgen:gateway_out_config  block_width_w=590  block_height_w=620  block_width=620  block_height=750
  Mult : hdlBasic/Mult  precision=User Defined  arith_type="Signed  (2's comp)"  n_bits=mu_mult_ni  bin_pt=mu_mult_nf  quantization="Round  (unbiased: +/- Inf)"  overflow=Wrap  en=off  latency=2  opt_float=off  fp_mult_usage=No Usage  use_behavioral_HDL=off  opt=Speed  use_embedded=on  optimum_pipeline=off  pipeline=off  use_rpm=off  placement_style=Rectangular shape  XmcBlockStatus=1  maskContainerNames=group1  block_type=mult  block_config=sysgen:Mult_config  block_width=598  block_height=876
  Mult1 : hdlBasic/Mult  precision=User Defined  arith_type="Signed  (2's comp)"  n_bits=mu_mult_ni  bin_pt=mu_mult_nf  quantization="Round  (unbiased: +/- Inf)"  overflow=Wrap  en=off  latency=2  opt_float=off  fp_mult_usage=No Usage  use_behavioral_HDL=off  opt=Speed  use_embedded=on  optimum_pipeline=off  pipeline=off  use_rpm=off  placement_style=Rectangular shape  XmcBlockStatus=1  maskContainerNames=group1  block_type=mult  block_config=sysgen:Mult_config  block_width=598  block_height=876
  Real-Imag to Complex2 : RealImagToComplex
  Sub1 : hdlBasic/AddSub  mode=Subtraction  use_carryin=off  use_carryout=off  en=off  latency=1  precision=User Defined  arith_type="Signed  (2's comp)"  n_bits=err_ni  bin_pt=err_nf  quantization=Truncate  overflow=Saturate  use_behavioral_HDL=on  hw_selection=Fabric  pipelined=off  use_rpm=off  XmcBlockStatus=1  maskContainerNames=tabcontainer1  block_type=addsub  block_config=sysgen:Addsub_config
  Sub2 : hdlBasic/AddSub  mode=Subtraction  use_carryin=off  use_carryout=off  en=off  latency=1  precision=User Defined  arith_type="Signed  (2's comp)"  n_bits=err_ni  bin_pt=err_nf  quantization="Round  (unbiased: +/- Inf)"  overflow=Saturate  use_behavioral_HDL=on  hw_selection=Fabric  pipelined=off  use_rpm=off  XmcBlockStatus=1  maskContainerNames=tabcontainer1  block_type=addsub  block_config=sysgen:Addsub_config
  mu : hdlBasic/Constant  const=mu  gui_display_data_type=Fixed-point  arith_type=Signed (2's comp)  n_bits=mu_ni  bin_pt=mu_nf  preci_type=Single  exp_width=8  frac_width=24  explicit_period=off  period=1  XmcBlockStatus=1  maskContainerNames=tabcontainer1  block_type=constant  block_config=sysgen:Constant_config
  neg_mu : hdlBasic/Constant  const=-mu  gui_display_data_type=Fixed-point  arith_type=Signed (2's comp)  n_bits=mu_ni  bin_pt=mu_nf  preci_type=Single  exp_width=8  frac_width=24  explicit_period=off  period=1  XmcBlockStatus=1  maskContainerNames=tabcontainer1  block_type=constant  block_config=sysgen:Constant_config
  muErr_I : Outport  VectorParamsAs1DForOutWhenUnconnected=off
  muErr_Q : Outport  Port=2  VectorParamsAs1DForOutWhenUnconnected=off
  err_n : Outport  Port=3  VectorParamsAs1DForOutWhenUnconnected=off
  wires:
  Mult/1 -> muErr_I/1
  Mult1/1 -> muErr_Q/1
  neg_mu/1 -> Mult1/2
  mu/1 -> Mult/2
  det_I/1 -> Sub1/1
  dhat_I/1 -> Sub1/2
  det_Q/1 -> Sub2/1
  dhat_Q/1 -> Sub2/2
  Sub1/1 -> Mult/1, Gateway Out4/1
  Sub2/1 -> Mult1/1, Gateway Out5/1
  Real-Imag to Complex2/1 -> err_n/1
  Gateway Out4/1 -> Real-Imag to Complex2/1
  Gateway Out5/1 -> Real-Imag to Complex2/2

== system QAM16/DUT/Carrier Recovery/Cmplx Mult ==
  a_r : Inport
  a_i : Inport  Port=2
  b_r : Inport  Port=3
  b_i : Inport  Port=4
  AddSub : hdlBasic/AddSub  mode=Subtraction  use_carryin=off  use_carryout=off  en=off  latency=0  precision=User Defined  arith_type="Signed  (2's comp)"  n_bits=lms_mult_post_add_ni  bin_pt=lms_mult_post_add_nf  quantization=Truncate  overflow=Wrap  use_behavioral_HDL=on  hw_selection=Fabric  pipelined=off  use_rpm=on  XmcBlockStatus=1  maskContainerNames=tabcontainer1  block_type=addsub  block_config=sysgen:Addsub_config
  AddSub1 : hdlBasic/AddSub  mode=Addition  use_carryin=off  use_carryout=off  en=off  latency=0  precision=User Defined  arith_type="Signed  (2's comp)"  n_bits=lms_mult_post_add_ni  bin_pt=lms_mult_post_add_nf  quantization=Truncate  overflow=Wrap  use_behavioral_HDL=on  hw_selection=Fabric  pipelined=off  use_rpm=on  XmcBlockStatus=1  maskContainerNames=tabcontainer1  block_type=addsub  block_config=sysgen:Addsub_config
  Mult{1..4} (4 alike) : hdlBasic/Mult  precision=User Defined  arith_type="Signed  (2's comp)"  n_bits=lms_mult_ni  bin_pt=lms_mult_nf  quantization=Truncate  overflow=Wrap  en=off  latency=0  opt_float=off  fp_mult_usage=No Usage  use_behavioral_HDL=off  opt=Speed  use_embedded=on  optimum_pipeline=off  pipeline=off  use_rpm=on  placement_style=Rectangular shape  XmcBlockStatus=1  maskContainerNames=group1  block_type=mult  block_config=sysgen:Mult_config  block_width=598  block_height=876
  p_r : Outport  VectorParamsAs1DForOutWhenUnconnected=off
  p_i : Outport  Port=2  VectorParamsAs1DForOutWhenUnconnected=off
  wires:
  AddSub1/1 -> p_i/1
  AddSub/1 -> p_r/1
  Mult3/1 -> AddSub1/2
  Mult2/1 -> AddSub1/1
  Mult1/1 -> AddSub/2
  a_r/1 -> Mult2/1, Mult4/1
  b_i/1 -> Mult2/2, Mult1/2
  b_r/1 -> Mult3/1, Mult4/2
  a_i/1 -> Mult3/2, Mult1/1
  Mult4/1 -> AddSub/1

== system QAM16/DUT/Carrier Recovery/Cmplx Mult1 ==
  a_r : Inport
  a_i : Inport  Port=2
  b_r : Inport  Port=3
  b_i : Inport  Port=4
  AddSub : hdlBasic/AddSub  mode=Subtraction  use_carryin=off  use_carryout=off  en=off  latency=0  precision=User Defined  arith_type="Signed  (2's comp)"  n_bits=lms_mult_post_add_ni  bin_pt=lms_mult_post_add_nf  quantization=Truncate  overflow=Wrap  use_behavioral_HDL=on  hw_selection=Fabric  pipelined=off  use_rpm=on  XmcBlockStatus=1  maskContainerNames=tabcontainer1  block_type=addsub  block_config=sysgen:Addsub_config
  AddSub1 : hdlBasic/AddSub  mode=Addition  use_carryin=off  use_carryout=off  en=off  latency=0  precision=User Defined  arith_type="Signed  (2's comp)"  n_bits=lms_mult_post_add_ni  bin_pt=lms_mult_post_add_nf  quantization=Truncate  overflow=Wrap  use_behavioral_HDL=on  hw_selection=Fabric  pipelined=off  use_rpm=on  XmcBlockStatus=1  maskContainerNames=tabcontainer1  block_type=addsub  block_config=sysgen:Addsub_config
  Mult{1..4} (4 alike) : hdlBasic/Mult  precision=User Defined  arith_type="Signed  (2's comp)"  n_bits=lms_mult_ni  bin_pt=lms_mult_nf  quantization=Truncate  overflow=Wrap  en=off  latency=0  opt_float=off  fp_mult_usage=No Usage  use_behavioral_HDL=off  opt=Speed  use_embedded=on  optimum_pipeline=off  pipeline=off  use_rpm=on  placement_style=Rectangular shape  XmcBlockStatus=1  maskContainerNames=group1  block_type=mult  block_config=sysgen:Mult_config  block_width=598  block_height=876
  p_r : Outport  VectorParamsAs1DForOutWhenUnconnected=off
  p_i : Outport  Port=2  VectorParamsAs1DForOutWhenUnconnected=off
  wires:
  Mult4/1 -> AddSub/1
  a_i/1 -> Mult1/1, Mult3/2
  b_r/1 -> Mult4/2, Mult3/1
  b_i/1 -> Mult1/2, Mult2/2
  a_r/1 -> Mult4/1, Mult2/1
  Mult1/1 -> AddSub/2
  Mult2/1 -> AddSub1/1
  Mult3/1 -> AddSub1/2
  AddSub/1 -> p_r/1
  AddSub1/1 -> p_i/1

== system QAM16/DUT/Carrier Recovery/DDS ==
  In1 : Inport
  In2 : Inport  Port=2
  Convert : hdlBasic/Convert  gui_display_data_type=Fixed-point  arith_type=Unsigned  n_bits=14  bin_pt=14  float_type=Single  exp_bits=8  fraction_bits=24  quantization=Truncate  overflow=Wrap  en=off  latency=0  pipeline=off  XmcBlockStatus=1  maskContainerNames=group2  block_type=convert  block_config=sysgen:Convert_config  block_width=595  block_height=885
  "DDS Compiler 6.0 " : hdlDSPIP/DDS Compiler 6.0   partspresent=Phase_Generator_and_SIN_COS_LUT  dds_clock_rate=100  channels=1  mode_of_operation=Standard  output_type=Integer  modulus=9  parameter_entry=System_Parameters  spurious_free_dynamic_range=96  frequency_resolution=10000  noise_shaping=Auto  phase_width=28  output_width=8  output_selection=Sine_and_Cosine  negative_sine=off  negative_cosine=off  amplitude_mode=Full_Range  memory_type=Auto  optimization_goal=Auto  dsp48_use=Minimal  resync=off  latency_configuration=Auto  latency=7  has_phase_out=off  has_aclken=off  has_aresetn=off  explicit_period=off  period=1  data_has_tlast=Not_Required  has_tready=off  s_phase_has_tuser=Not_Required  m_data_has_tuser=Not_Required  m_phase_has_tuser=Not_Required  s_phase_tuser_width=1  output_form=Twos_Complement  s_config_sync_mode=On_Vector  phase_increment=Programmable  output_frequency1=0  output_frequency2=0  output_frequency3=0  output_frequency4=0  output_frequency5=0  output_frequency6=0  output_frequency7=0  output_frequency8=0  output_frequency9=0  output_frequency10=0  output_frequency11=0  output_frequency12=0  output_frequency13=0  output_frequency14=0  output_frequency15=0  output_frequency16=0  pinc1='1101000110110111'  pinc2='0'  pinc3='0'  pinc4='0'  pinc5='0'  pinc6='0'  pinc7='0'  pinc8='0'  pinc9='0'  pinc10='0'  pinc11='0'  pinc12='0'  pinc13='0'  pinc14='0'  pinc15='0'  pinc16='0'  phase_offset=None  phase_offset_angles1=0  phase_offset_angles2=0  phase_offset_angles3=0  phase_offset_angles4=0  phase_offset_angles5=0  phase_offset_angles6=0  phase_offset_angles7=0  phase_offset_angles8=0  phase_offset_angles9=0  phase_offset_angles10=0  phase_offset_angles11=0  phase_offset_angles12=0  phase_offset_angles13=0  phase_offset_angles14=0  phase_offset_angles15=0  phase_offset_angles16=0  poff1='0'  poff2='0'  poff3='0'  poff4='0'  poff5='0'  poff6='0'  poff7='0'  poff8='0'  poff9='0'  poff10='0'  poff11='0'  poff12='0'  poff13='0'  poff14='0'  poff15='0'  poff16='0'  trim_axipin_name=on  simulation_type=hybrid_sim  simulation_model=sysgen:xddsv6_0_cmodel  data_path_portlist={ 's_axis_config_tdata_poff', 's_axis_config_tdata_chan0_poff', 's_axis_config_tdata_pinc', 's_axis_config_tdata_chan0_pinc', 's_axis_phase_tdata_resync', 's_axis_phase_tdata_chan0_resync', 's_axis_phase_tdata_poff', 's_axis_phase_tdata_chan0_poff', 's_axis_phase_tdata_pinc', 's_axis_phase_tdata_chan0_pinc', 's_axis_phase_tdata_phase_in', 'm_axis_data_tdata_sine', 'm_axis_data_tdata_chan0_sine', 'm_axis_data_tdata_cosine', 'm_axis_data_tdata_chan0_cosine', 'm_axis_phase_tdata_phase_out', 'm_axis_phase_tdata_chan0_phase_out'}  por_mode=false  gui_behaviour=Sysgen  ip_name=DDS Compiler  ip_version=6.0  dsptool_ready=true  wrapper_available=true  port_translation_map={ 'aclken' => 'en', 'aresetn' => 'rst' }  ipcore_usecache=true  ipcore_useipmodelcache=true  ipcore_xco_need_fpga_part=true  ipcore_fpga_part=xlipgetpartsetting(gcb, {'virtex7', 'xc7v1500t', '-2', 'fhg1157'})  ipcore_verbose=false  XmcBlockStatus=1  maskContainerNames=tabcontainer1  block_type=dds_compiler_v6_0  block_config=sysgen:rodinimport_config  block_width=760
  Register : hdlBasic/Register  init=0  rst=off  en=on  XmcBlockStatus=1  maskContainerNames=tabcontainer1  block_type=register  block_config=sysgen:Register_config
  Register1 : hdlBasic/Register  init=0  rst=off  en=on  XmcBlockStatus=1  maskContainerNames=tabcontainer1  block_type=register  block_config=sysgen:Register_config
  Reinterpret : hdlBasic/Reinterpret  force_arith_type=on  arith_type="Signed  (2's comp)"  force_bin_pt=off  bin_pt=0  XmcBlockStatus=1  maskContainerNames=group1  block_type=cast  block_config=sysgen:Reinterpret_config
  Reinterpret1 : hdlBasic/Reinterpret  force_arith_type=off  arith_type="Signed  (2's comp)"  force_bin_pt=on  bin_pt=15  XmcBlockStatus=1  maskContainerNames=group1  block_type=cast  block_config=sysgen:Reinterpret_config
  Reinterpret2 : hdlBasic/Reinterpret  force_arith_type=off  arith_type="Signed  (2's comp)"  force_bin_pt=on  bin_pt=15  XmcBlockStatus=1  maskContainerNames=group1  block_type=cast  block_config=sysgen:Reinterpret_config
  Reinterpret3 : hdlBasic/Reinterpret  force_arith_type=on  arith_type=Unsigned  force_bin_pt=off  bin_pt=0  XmcBlockStatus=1  maskContainerNames=group1  block_type=cast  block_config=sysgen:Reinterpret_config
  Out1 : Outport  VectorParamsAs1DForOutWhenUnconnected=off
  Out2 : Outport  Port=2  VectorParamsAs1DForOutWhenUnconnected=off
  wires:
  In1/1 -> Convert/1
  Convert/1 -> Reinterpret/1
  Register/1 -> Reinterpret2/1
  Register1/1 -> Reinterpret1/1
  Reinterpret2/1 -> Out1/1
  Reinterpret1/1 -> Out2/1
  "DDS Compiler 6.0 "/2 -> Register/1
  "DDS Compiler 6.0 "/3 -> Register1/1
  Reinterpret/1 -> Reinterpret3/1
  In2/1 -> "DDS Compiler 6.0 "/1
  "DDS Compiler 6.0 "/1 -> Register/2, Register1/2
  Reinterpret3/1 -> "DDS Compiler 6.0 "/2
